simulink library "dspmlti4"  (Simulink 6.0)
settings: Solver=ode45  SolverMode=SingleTasking  StartTime=0.0  StopTime=10.0  RelTol=1e-3
undefined symbols (not defined in the file or in its folder): Hm_decim, Hm_interp, remez
libraries: dspmlti3 x3, simulink x1
settings Model: RequirementInfo=9  CovMetricSettings=d  Creator=tbryan  LastModifiedBy=sconahan  ExtModeAutoUpdateStatusClock=off  ProdHWDeviceType=Specified
settings DataIOCC: SignalLoggingName=logsOut
settings OptimizationCC: BooleanDataType=off
settings DebuggingCC: CheckExecutionContextPreStartOutputMsg=on  CheckExecutionContextRuntimeOutputMsg=on  SolverPrmCheckMsg=none
settings HardwareCC: ProdHWDeviceType=Specified  TargetUnknown=on
settings SFSimCC: SFSimApplyToAllLibs=on  SFSimBuildMode=Incremental

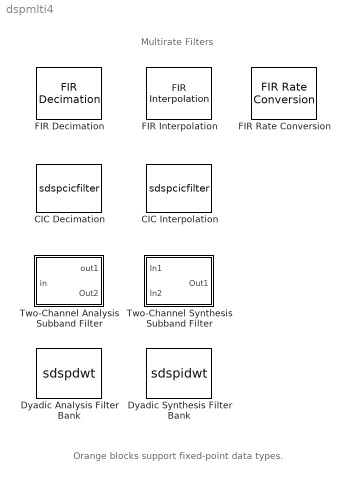
== system dspmlti4 ==
  note: Multirate Filters
  note: Orange blocks support
      | fixed-point data types.
  CIC Decimation : S-Function  FunctionName=sdspcicfilter  Parameters=ftype_Sfcn, R_Sfcn, M_Sfcn, N_Sfcn, stage2NWL_Sfcn, outWL_Sfcn, states_Sfcn, resampPhase_Sfcn, framing  mask(CIC Decimation){filtFrom=Dialog, filtobj=Hm_decim, ftype=Decimator, R=2, resampPhase=0, M=1, N=2, BPS=[16 16 16 16], outputMode=Same as final filter stage, outputWordLength=32, launchFVT=off, framing=Maintain input frame rate}
      mask prompts: filtFrom "Filter specified via:"; filtobj "Multirate filter variable:"; ftype "Filter structure:"; R "Decimation factor (R):"; resampPhase "Resampler phase (0 to R-1):"; M "Differential delay (M):"; N "Number of stages (N):"; BPS "Word length for each of the (2*N) filter stages:"; outputMode "Output word length mode:"; outputWordLength "Output word length:"; launchFVT "Launch Filter Visualization Tool (FVTool)"
      mask help:
      | Apply a Cascaded Integrator-Comb Decimator filter to the input signal. You can define the filter with the mask parameters, or by a CIC multirate filter (MFILT) object defined in the MATLAB workspace. You can use the latter option only when the Filter Design Toolbox is installed.
      |
      | When you choose a filter structure with zero latency, the filter output is not delayed. The outputs of the other structures are delayed by N.
      |
      | Inputs and outputs are signed fixed-point data types with zero bias.  Output scaling is inherited from the input.
      mask init:
      | [ftype_Sfcn, R_Sfcn, M_Sfcn, N_Sfcn, stage2NWL_Sfcn, outWL_Sfcn, states_Sfcn, resampPhase_Sfcn] = dspblkcicfilter('init',R,resampPhase,M,N,BPS,outputWordLength,filtobj);
      settings: CopyFcn=dspfixptcopycallback
      mask StyleString: popup(Dialog|Multirate object in workspace),edit,popup(Decimator|Zero-latency decimator),edit,edit,edit,edit,edit,popup(Same as final filter stage|Same as input|User-defined),edit,checkbox,popup(Maintain input frame rate|Maintain input frame size)
      mask CallbackString: dspblkcicfilter('dynamic');||dspblkcicfilter('dynamic');||||||dspblkcicfilter('dynamic');||dspblkcicfilter('dynamic',get_param(gcb,'launchFVT'));|
      mask Display: disp(dspblkcicfilter('icon'));
  CIC Interpolation : S-Function  FunctionName=sdspcicfilter  Parameters=ftype_Sfcn, R_Sfcn, M_Sfcn, N_Sfcn, stage2NWL_Sfcn, outWL_Sfcn, states_Sfcn, resampPhase_Sfcn, framing  mask(CIC Interpolation){filtFrom=Dialog, filtobj=Hm_interp, ftype=Interpolator, R=2, resampPhase=0, M=1, N=2, filtStageWLMode=Use minimum number of bits per stage, BPS=[16 16 16 16], outputMode=Same as final filter stage, outputWordLength=32, launchFVT=off, framing=Maintain input frame rate}
      mask prompts: filtFrom "Filter specified via:"; filtobj "Multirate filter variable:"; ftype "Filter structure:"; R "Interpolation factor (R):"; resampPhase "Resampler phase (0 to R-1):"; M "Differential delay (M):"; N "Number of stages (N):"; filtStageWLMode "Filter stages word length mode:"; BPS "Word length for each of the (2*N) filter stages:"; outputMode "Output word length mode:"; outputWordLength "Output word length:"; launchFVT "Launch Filter Visualization Tool (FVTool)"
      mask help:
      | Apply a Cascaded Integrator-Comb Interpolator filter to the input signal. You can define the filter with the mask parameters, or by a CIC multirate filter (MFILT) object defined in the MATLAB workspace. You can use the latter option only when the Filter Design Toolbox is installed.
      |
      | When you choose a filter structure with zero latency, the filter output is not delayed. The outputs of the other structures are delayed by N.
      |
      | Inputs and outputs are signed fixed-point data types with zero bias.  Output scaling is inherited from the input.
      mask init:
      | if (strcmpi(get_param(gcb,'filtFrom'),'Dialog') && strcmpi(get_param(gcb,'filtStageWLMode'),'Use minimum number of bits per stage')),
      | 	BPS_mask_helper = -1;
      | else
      | 	BPS_mask_helper = BPS;
      | end
      | [ftype_Sfcn, R_Sfcn, M_Sfcn, N_Sfcn, stage2NWL_Sfcn, outWL_Sfcn, states_Sfcn, resampPhase_Sfcn] = dspblkcicfilter('init',R,resampPhase,M,N,BPS_mask_helper,outputWordLength,filtobj);
      settings: CopyFcn=dspfixptcopycallback
      mask StyleString: popup(Dialog|Multirate object in workspace),edit,popup(Interpolator|Zero-latency interpolator),edit,edit,edit,edit,popup(Use minimum number of bits per stage|User-defined),edit,popup(Same as final filter stage|Same as input|User-defined),edit,checkbox,popup(Maintain input frame rate|Maintain input frame size)
      mask CallbackString: dspblkcicfilter('dynamic');||dspblkcicfilter('dynamic');|||||dspblkcicfilter('dynamic');||dspblkcicfilter('dynamic');||dspblkcicfilter('dynamic',get_param(gcb,'launchFVT'));|
      mask Display: disp(dspblkcicfilter('icon'));
  Dyadic Analysis Filter Bank : S-Function  FunctionName=sdspdwt  Parameters=phl, phh, NumLevels, tree, Output  mask(Dyadic Analysis Filter Bank){Wname=User-defined, OrdRec_ordDec=[1 / 1], Order=2, LPF=[0.0352   -0.0854   -0.1350   0.4599   0.8069   0.3327], HPF=[-0.3327    0.8069   -0.4599   -0.1350    0.0854    0.0352], NumLevels=2, tree=Asymmetric, Output=Multiple ports}
      mask prompts: Wname "Filter:"; OrdRec_ordDec "Filter order [synthesis / analysis]:"; Order "Wavelet order:"; LPF "Lowpass FIR filter coefficients:"; HPF "Highpass FIR filter coefficients:"; NumLevels "Number of levels:"; tree "Tree structure:"
      mask help:
      | Decomposes a signal into subbands with smaller bandwidths and slower sample rates. Uses a filter bank with specified lowpass and highpass FIR filters, which can be user-defined or wavelet-based (use of wavelets requires the Wavelet Toolbox). Usually, the lowpass and highpass filters should be half-band filters designed to complement each other.
      |
      |
      | When 'Output' is set to 'Multiple ports', the block outputs each subband from a different port as a frame-based vector or matrix (the topmost port outputs the subband with the highest frequency band). When 'Output' is set to 'Single port', the block outputs one sample-based vector or matrix of concatenated subbands.
      |
      |
      | Inputs must be frame-based with a frame size a multiple of 2^n, where n is the value entered in the 'Number of levels.'  To create a filter bank that accepts sample-based inputs and inputs of other sizes, use Two-Channel Analysis Subband Filter blocks in the Multirate Filters library.
      |
      |
      | This block is the same as the DWT block in the Transforms library.
      mask init:
      | [x,y, str] = dspblkdwt('icon');
      | [phl, phh] = dspblkdwt('init', LPF, HPF, tree);
      mask Help: web(dspbhelp);
      mask StyleString: popup(User-defined|Haar|Daubechies|Symlets|Coiflets|Biorthogonal|Reverse Biorthogonal|Discrete Meyer),popup([1 / 1]|[1 / 3]|[1 / 5]|[2 / 2]|[2 / 4]|[2 / 6]|[2 / 8]|[3 / 1]|[3 / 3]|[3 / 5]|[3 / 7]|[3 / 9]|[4 / 4]|[5 / 5]|[6 / 8]),edit,edit,edit,edit,popup(Asymmetric|Symmetric),popup(Single port|Multiple ports)
      mask CallbackString: dspblkdwt|||||||
      mask Display:
      | plot(x,y)
      | text(0.08,0.1,str)
  Dyadic Synthesis Filter Bank : S-Function  FunctionName=sdspidwt  Parameters=phl, phh, NumLevels, tree, Input  mask(Dyadic Synthesis Filter Bank){Wname=User-defined, OrdRec_ordDec=[1 / 1], Order=2, LPF=[0.3327    0.8069    0.4599   -0.1350   -0.0854    0.0352], HPF=[0.0352    0.0854   -0.1350   -0.4599    0.8069   -0.3327], NumLevels=2, tree=Asymmetric, Input=Multiple ports}
      mask prompts: Wname "Filter:"; OrdRec_ordDec "Filter order [synthesis, analysis]:"; Order "Wavelet order:"; LPF "Lowpass FIR filter coefficients:"; HPF "Highpass FIR filter coefficients:"; NumLevels "Number of levels:"; tree "Tree Structure:"
      mask help:
      | Reconstructs a signal from its subbands with smaller bandwidths and slower sample rates. Uses a filter bank with specified lowpass and highpass FIR filters, which can be user-defined or wavelet-based (use of wavelets requires the Wavelet Toolbox). Usually, the lowpass and highpass filters should be half-band filters designed to complement each other.
      |
      |
      | When 'Input' is set to 'Multiple ports', you must input each subband through a different input port as a frame-based vector or matrix (the topmost input port should receive the subband with the highest frequency band). When 'Input' is set to 'Single port', the block input must be a sample-based vector or matrix of concatenated subbands.
      |
      |
      | To create a filter bank with less constraints on whether the inputs are frame-based or sample-based, use Two-Channel Synthesis Subband Filter blocks in the Multirate Filters library.
      |
      |
      | This block is the same as the IDWT block in the Transforms library.
      mask init:
      | [x,y,str] = dspblkidwt('icon');
      | [phl, phh] = dspblkidwt('init', LPF, HPF, tree);
      mask Help: web(dspbhelp);
      mask StyleString: popup(User-defined|Haar|Daubechies|Symlets|Coiflets|Biorthogonal|Reverse Biorthogonal|Discrete Meyer),popup([1 / 1]|[1 / 3]|[1 / 5]|[2 / 2]|[2 / 4]|[2 / 6]|[2 / 8]|[3 / 1]|[3 / 3]|[3 / 5]|[3 / 7]|[3 / 9]|[4 / 4]|[5 / 5]|[6 / 8]),edit,edit,edit,edit,popup(Asymmetric|Symmetric),popup(Single port|Multiple ports)
      mask CallbackString: dspblkidwt|||||||
      mask Display:
      | plot(x,y)
      | text(0.08,0.1,str)
  FIR Decimation : dspmlti3/FIR Decimation  DialogController=dspDDGCreate  DialogControllerArgs=DataTag2  h=fir1(35,0.4)  D=2  framing=Maintain input frame size  outputBufInitCond=0  roundingMode=Floor  overflowMode=off
  FIR Interpolation : dspmlti3/FIR Interpolation  DialogController=dspDDGCreate  DialogControllerArgs=DataTag3  h=fir1(15,1/4)  L=3  framing=Maintain input frame size  outputBufInitCond=0  roundingMode=Floor  overflowMode=off
  FIR Rate Conversion : dspmlti3/FIR Rate Conversion  DialogController=dspDDGCreate  DialogControllerArgs=DataTag4  L=3  h=remez(70,[0 .28 .32 1],[1 1 0 0])  M=2  roundingMode=Floor  overflowMode=off
  Two-Channel Analysis Subband Filter : Subsystem  DialogController=dspDDGCreate  DialogControllerArgs=DataTag5  PropExecContextAcrossSSBoundary=on  mask(Two-Channel Analysis Subband Filter){lpf=[0.0352   -0.0854   -0.1350   0.4599   0.8069   0.3327], hpf=[-0.3327    0.8069   -0.4599   -0.1350    0.0854    0.0352], framing=Maintain input frame size, additionalParams=off, allowOverrides=off, firstCoeffMode=Same word length as input, firstCoeffWordLength=16, firstCoeffFracLength=15, outputMode=Same as accumulator, outputWordLength=16, outputFracLength=14, accumMode=Inherit via internal rule, accumWordLength=32, accumFracLength=30, prodOutputMode=Inherit via internal rule, prodOutputWordLength=32, prodOutputFracLength=30, roundingMode=Floor, overflowMode=off}
      mask prompts: lpf "Lowpass FIR filter coefficients:"; hpf "Highpass FIR filter coefficients:"; additionalParams "--------------- Show additional parameters ---------------"; allowOverrides "Allow overrides from DSP Fixed-Point Attributes blocks"; firstCoeffMode "Fixed-point coefficient attributes:"; firstCoeffWordLength "Coefficient word length:"; firstCoeffFracLength "Coefficient fraction length:"; outputMode "Fixed-point output attributes:"; outputWordLength "Output word length:"; outputFracLength "Output fraction length:"; accumMode "Fixed-point accumulator attributes:"; accumWordLength "Accumulator word length:"; accumFracLength "Accumulator fraction length:"; prodOutputMode "Fixed-point product output attributes:"; prodOutputWordLength "Product output word length:"; prodOutputFracLength "Product output fraction length:"; roundingMode "Round integer calculations towards:"; overflowMode "Saturate on integer overflow"
      mask help:
      | Decompose a signal into a high-frequency subband (Hi band) and a low-frequency subband (Lo band) using the specified highpass and lowpass FIR filters.  Each subband has half the bandwidth and half the sample rate of the original signal.  Usually, the highpass and lowpass filters should be half-band filters designed to complement each other. This block accepts sample- and frame-based inputs of all sizes.
      |
      |
      | To implement a multilevel filter bank that decomposes a signal into more than two subbands, use the Dyadic Analysis Filter Bank block in the Multirate Filters library (accepts only frame-based inputs of certain sizes).
      |
      | For some fixed-point modes, the FIR filter coefficients fraction length or slope is automatically set for you to ''Best precision.'' In these cases, the scaling is set to the best possible precision given the real-world values and word length of the coefficients. This is equivalent to the ''Best Precision: Matrix-wise'' scaling option used in some Simulink fixed-point blocks.
      mask init:
      | outputBufInitCond = 0;
      | hpf    = dspblkfirdn2('setup',hpf,2);
      | lpf    = dspblkfirdn2('setup',lpf,2);
      | dtInfo = dspGetFixptDataTypeInfo(gcbh,47);
      settings: CopyFcn=dspfixptcopycallback
      mask Help: web(dspbhelp);
      mask StyleString: edit,edit,popup(Maintain input frame size|Maintain input frame rate),checkbox,checkbox,popup(Same word length as input|Specify word length|Binary point scaling|Slope and bias scaling|User-defined),edit,edit,popup(Same as accumulator|Same as product output|Same as input|Binary point scaling|Slope and bias scaling|User-defined),edit,edit,popup(Inherit via internal rule|Same as product output|Same as input|Binary point scaling|Slope and bias scaling|User-defined),edit,edit,popup(Inherit via internal rule|Same as input|Binary point scaling|Slope and bias scaling|User-defined),edit,edit,popup(Floor|Nearest),checkbox
      mask Display:
      | disp('');
      | port_label('output', 1, 'Hi band');
      | port_label('output', 2, 'Lo band');
  Two-Channel Synthesis Subband Filter : Subsystem  DialogController=dspDDGCreate  DialogControllerArgs=DataTag6  PropExecContextAcrossSSBoundary=on  mask(Two-Channel Synthesis Subband Filter){lpf=[0.3327    0.8069    0.4599   -0.1350   -0.0854    0.0352], hpf=[0.0352    0.0854   -0.1350   -0.4599    0.8069   -0.3327], framing=Maintain input frame size, additionalParams=off, allowOverrides=off, firstCoeffMode=Same word length as input, firstCoeffWordLength=16, firstCoeffFracLength=15, outputMode=Same as accumulator, outputWordLength=16, outputFracLength=14, accumMode=Inherit via internal rule, accumWordLength=32, accumFracLength=30, prodOutputMode=Inherit via internal rule, prodOutputWordLength=32, prodOutputFracLength=30, roundingMode=Floor, overflowMode=off}
      mask prompts: lpf "Lowpass FIR filter coefficients:"; hpf "Highpass FIR filter coefficients:"; additionalParams "--------------- Show additional parameters ---------------"; allowOverrides "Allow overrides from DSP Fixed-Point Attributes blocks"; firstCoeffMode "Fixed-point coefficient attributes:"; firstCoeffWordLength "Coefficient word length:"; firstCoeffFracLength "Coefficient fraction length:"; outputMode "Fixed-point output attributes:"; outputWordLength "Output word length:"; outputFracLength "Output fraction length:"; accumMode "Fixed-point accumulator attributes:"; accumWordLength "Accumulator word length:"; accumFracLength "Accumulator fraction length:"; prodOutputMode "Fixed-point product output attributes:"; prodOutputWordLength "Product output word length:"; prodOutputFracLength "Product output fraction length:"; roundingMode "Round integer calculations towards:"; overflowMode "Saturate on integer overflow"
      mask help:
      | Reconstruct a signal from a high-frequency subband (Hi band) and a low-frequnecy subband (Lo band) using the specified highpass and lowpass FIR filters.  The input subbands should have the same bandwidths and sample rates. Usually, the highpass and lowpass filters should be half-band filters designed to complement each other.  This block accepts sample- and frame-based inputs of all sizes.
      |
      |
      | To create a multilevel filter bank that reconstructs a signal from more than two subbands, use the Dyadic Synthesis Filter Bank block in the Multirate Filters library (has more constraints on its inputs).
      |
      | For some fixed-point modes, the FIR filter coefficients fraction length or slope is automatically set for you to ''Best precision.'' In these cases, the scaling is set to the best possible precision given the real-world values and word length of the coefficients. This is equivalent to the ''Best Precision: Matrix-wise'' scaling option used in some Simulink fixed-point blocks.
      mask init:
      | outputBufInitCond        = 0;
      | [hpf,outputBufInitCondH] = dspblkupfir2('setup',hpf,2,outputBufInitCond);
      | [lpf,outputBufInitCondL] = dspblkupfir2('setup',lpf,2,outputBufInitCond);
      | dtInfo                   = dspblk2chsbank('init');
      settings: CopyFcn=dspfixptcopycallback
      mask Help: web(dspbhelp);
      mask StyleString: edit,edit,popup(Maintain input frame size|Maintain input frame rate),checkbox,checkbox,popup(Same word length as input|Specify word length|Binary point scaling|Slope and bias scaling|User-defined),edit,edit,popup(Same as accumulator|Same as product output|Same as input|Binary point scaling|Slope and bias scaling|User-defined),edit,edit,popup(Inherit via internal rule|Same as product output|Same as input|Binary point scaling|Slope and bias scaling|User-defined),edit,edit,popup(Inherit via internal rule|Same as input|Binary point scaling|Slope and bias scaling|User-defined),edit,edit,popup(Floor|Nearest),checkbox
      mask Display:
      | disp('');
      | port_label('input', 1, 'Hi band');
      | port_label('input', 2, 'Lo band');

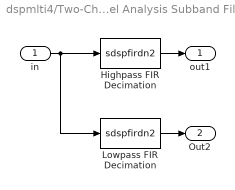
== system dspmlti4/Two-Channel Analysis Subband Filter ==
  in : Inport  LatchInput=off
  Highpass FIR Decimation : S-Function  FunctionName=sdspfirdn2  Parameters=hpf,2,framing,outputBufInitCond,dtInfo.firstCoeffMode,dtInfo.firstCoeffWordLength,dtInfo.firstCoeffFracLength,dtInfo.prodOutputMode,dtInfo.prodOutputWordLength,dtInfo.prodOutputFracLength,dtInfo.accumMode,dtInfo.accumWordLength,dtInfo.accumFracLength,dtInfo.outputMode,dtInfo.outputWordLength,dtInfo.outputFracLength,dtInfo.roundingMode,dtInfo.overflowMode
  Lowpass FIR Decimation : S-Function  FunctionName=sdspfirdn2  Parameters=lpf,2,framing,outputBufInitCond,dtInfo.firstCoeffMode,dtInfo.firstCoeffWordLength,dtInfo.firstCoeffFracLength,dtInfo.prodOutputMode,dtInfo.prodOutputWordLength,dtInfo.prodOutputFracLength,dtInfo.accumMode,dtInfo.accumWordLength,dtInfo.accumFracLength,dtInfo.outputMode,dtInfo.outputWordLength,dtInfo.outputFracLength,dtInfo.roundingMode,dtInfo.overflowMode
  out1 : Outport
  Out2 : Outport  Port=2
  wires:
  Highpass FIR Decimation/1 -> out1/1
  in/1 -> Lowpass FIR Decimation/1, Highpass FIR Decimation/1
  Lowpass FIR Decimation/1 -> Out2/1

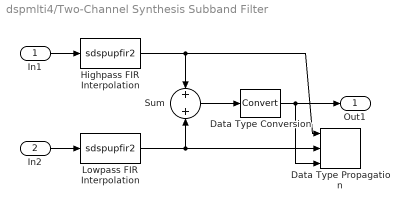
== system dspmlti4/Two-Channel Synthesis Subband Filter ==
  In1 : Inport  LatchInput=off
  In2 : Inport  Port=2  LatchInput=off
  Data Type Conversion : DataTypeConversion
  Data Type Propagation : simulink/Signal Attributes/Data Type Propagation  PropDataType=sfix(16)  IfRefDouble=double  IfRefSingle=single  IsSigned=IsSigned1 or IsSigned2  NumBitsBase=NumBits1  NumBitsMult=1  NumBitsAdd=0  NumBitsAllowFinal=1:128  PropScaling=2^-10  ValuesUsedBestPrec=[5 -7]  SlopeBase=Slope1  SlopeMult=1  SlopeAdd=0  BiasBase=Bias1  BiasMult=1  BiasAdd=0
  Highpass FIR Interpolation : S-Function  FunctionName=sdspupfir2  Parameters=hpf,2,framing,outputBufInitCondH,dtInfo.firstCoeffMode,dtInfo.firstCoeffWordLength,dtInfo.firstCoeffFracLength,dtInfo.prodOutputMode,dtInfo.prodOutputWordLength,dtInfo.prodOutputFracLength,dtInfo.accumMode,dtInfo.accumWordLength,dtInfo.accumFracLength,dtInfo.outputMode,dtInfo.outputWordLength,dtInfo.outputFracLength,dtInfo.roundingMode,dtInfo.overflowMode
  Lowpass FIR Interpolation : S-Function  FunctionName=sdspupfir2  Parameters=lpf,2,framing,outputBufInitCondL,dtInfo.firstCoeffMode,dtInfo.firstCoeffWordLength,dtInfo.firstCoeffFracLength,dtInfo.prodOutputMode,dtInfo.prodOutputWordLength,dtInfo.prodOutputFracLength,dtInfo.accumMode,dtInfo.accumWordLength,dtInfo.accumFracLength,dtInfo.outputMode,dtInfo.outputWordLength,dtInfo.outputFracLength,dtInfo.roundingMode,dtInfo.overflowMode
  Sum : Sum  Inputs=+|+  InputSameDT=on
  Out1 : Outport
  wires:
  In2/1 -> Lowpass FIR Interpolation/1
  Sum/1 -> Data Type Conversion/1
  In1/1 -> Highpass FIR Interpolation/1
  Lowpass FIR Interpolation/1 -> Data Type Propagation/2, Sum/2
  Highpass FIR Interpolation/1 -> Data Type Propagation/1, Sum/1
  Data Type Conversion/1 -> Out1/1, Data Type Propagation/3
